simulink model "simulink_laba_2_LV"  (R2023b)
settings: Solver=VariableStepAuto  StartTime=0.0  StopTime=20.0  RelTol=1e-3
settings Model: SnapshotBufferSize=20  SnapshotInterval=1  Creator=dimon  LastModifiedBy=dimon

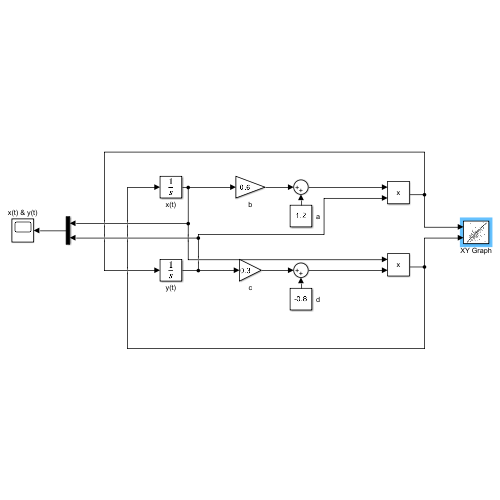
[thumbnail: Simulink's stored preview of the top-level diagram]
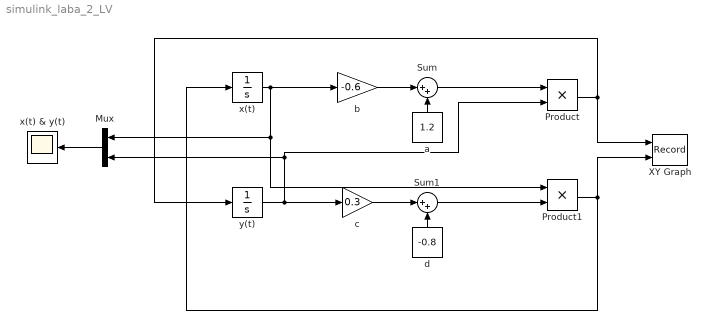
== system simulink_laba_2_LV ==
  Mux : Mux  Inputs=2
  Product : Product
  Product1 : Product
  Sum : Sum  Inputs=|++
  Sum1 : Sum  Inputs=|++
  XY Graph : Record  FileSettingsInternal="{\"entries\":[{\"content\":{\"excelSettings\":{\"content\":{},\"type\":\"Streamout.ExcelSettings\"}},\"type\":\"Streamout.FileSettingStorage\",\"uuid\":\"\"}],\"packageUris\":[\"http:\\/\\/schema.mathworks.com\\/mf0\\/streamout_blocks\\/R2020a\"],\"version\":\"1.0\"}"  Layout=[1 1]  SignalsInternal="{\"entries\":[{\"content\":{\"signals\":[{\"content\":{\"blockPath\":[],\"dimensions\":[1],\"domain\":\"\",\"lineColor\":\"#a2142f\",\"plots\":[ 1 ],\"port\":1,\"sid\":[\"\"],\"signalID\":1,\"signalName\":\"Product\"},\"type\":\"RecordBlkView.Signal\",\"uuid\":\"\"},{\"content\":{\"blockPath\":[],\"dimensions\":[1],\"domain\":\"\",\"lineColor\":\"#139fff\",\"plots\":[ 1 ],\"port\":2,\"sid\":[\"\"],\"signalID\":2,\"signalName\":\"Product1\"},\"type\":\"RecordBlkView.Signal\",\"uuid\":\"\"}]},\"type\":\"RecordBlkView.InputSignals\",\"uuid\":\"\"}],\"packageUris\":[\"http:\\/\\/schema.mathworks.com\\/mf0\\/streamout_blocks\\/R2020a\"],\"version\":\"1.0\"}"  VisualizationBindings="{\"xyplotplugin\":{\"info\":[{\"series\":[{\"bindingParametersList\":[{\"parameter\":\"X-Axis\",\"signalID\":1,\"signalName\":\"Product\"},{\"parameter\":\"Y-Axis\",\"signalID\":2,\"signalName\":\"Product1\"}],\"seriesID\":0}],\"subplotID\":1}]}}"  CompatibilityTag=XY
  a : Constant  Value=1.2
  b : Gain  Gain=-0.6
  d : Constant  Value=-0.8
  x(t) : Integrator  InitialCondition=2
  x(t) & y(t) : Scope
  y(t) : Integrator  InitialCondition=1
  с : Gain  Gain=0.3
  wires:
  x(t)/1 -> b/1, Mux/1, Product1/1
  a/1 -> Sum/2
  b/1 -> Sum/1
  Sum/1 -> Product/1
  y(t)/1 -> с/1, Product/2, Mux/2
  с/1 -> Sum1/1
  d/1 -> Sum1/2
  Sum1/1 -> Product1/2
  Product/1 -> XY Graph/1, y(t)/1
  Product1/1 -> XY Graph/2, x(t)/1
  Mux/1 -> x(t) & y(t)/1
